simulink model "uav_ue4_depth_imaging"  (R2021b)
settings: Solver=VariableStepAuto  StartTime=0.0  StopTime=10.0  RelTol=1e-3
libraries: visionsinks x3, sim3dcameralib x1, sim3dlib x1, uavsim3dlib x1, simulink x1
settings Model: Creator=The MathWorks, Inc.  LastModifiedBy=The MathWorks, Inc.
settings SolverCC: AlgebraicLoopSolver=TrustRegion
settings DebuggingCC: SFMachineParentedDataDiag=warning

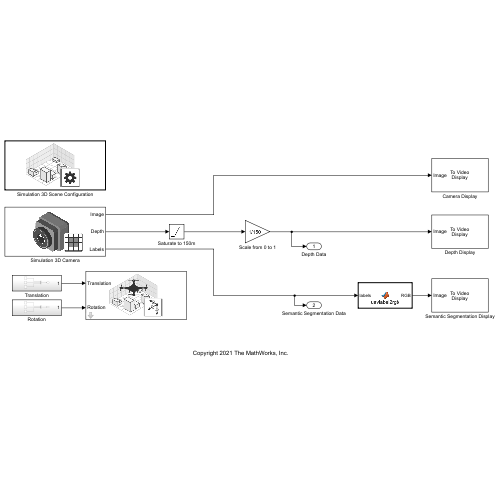
[thumbnail: Simulink's stored preview of the top-level diagram]
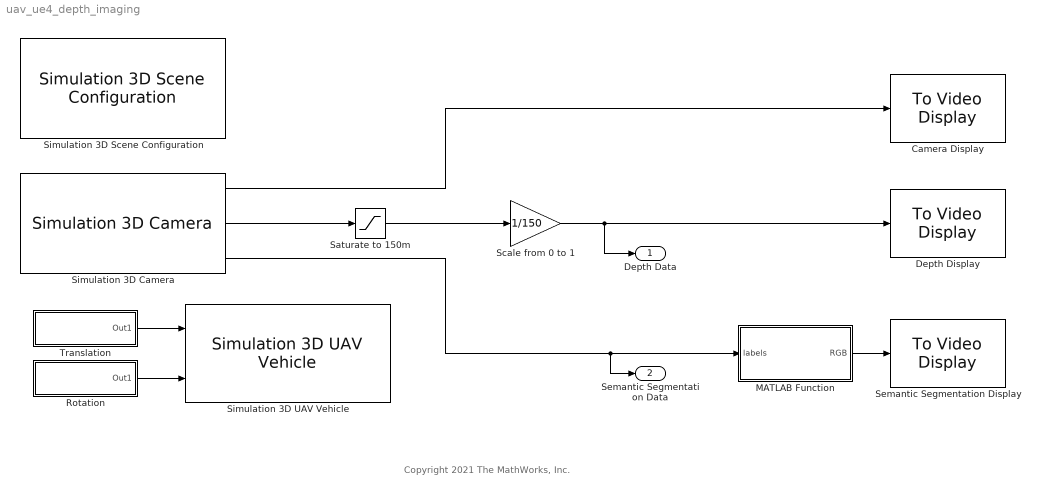
== system uav_ue4_depth_imaging ==
  note: Copyright 2021 The MathWorks, Inc.
  Camera Display : visionsinks/To Video Display  windowSizeMode=Normal  openAtMdlStart=on  fullScreen=off  videoWindowX=3778  videoWindowY=476  saveWindowSize=off  videoWindowWidth=1280  videoWindowHeight=720  inputColorFormat=RGB  inputType=Obsolete  imagePorts=One multidimensional signal  OutputDevice=On-screen video monitor  dataOrg=Column-major  isWindowOpen=off
  Depth Display : visionsinks/To Video Display  windowSizeMode=Normal  openAtMdlStart=on  fullScreen=off  videoWindowX=2800  videoWindowY=206  saveWindowSize=off  videoWindowWidth=1280  videoWindowHeight=720  inputColorFormat=RGB  inputType=Obsolete  imagePorts=One multidimensional signal  OutputDevice=On-screen video monitor  dataOrg=Column-major  isWindowOpen=off
  MATLAB Function : MATLAB Function  TreatAsAtomicUnit=on
  Rotation : Subsystem
  Saturate to 150m : Saturate  UpperLimit=150  LowerLimit=0
  Scale from 0 to 1 : Gain  Gain=1/150
  Semantic Segmentation Display : visionsinks/To Video Display  windowSizeMode=Normal  openAtMdlStart=on  fullScreen=off  videoWindowX=2682  videoWindowY=595  saveWindowSize=off  videoWindowWidth=1280  videoWindowHeight=720  inputColorFormat=RGB  inputType=Obsolete  imagePorts=One multidimensional signal  OutputDevice=On-screen video monitor  dataOrg=Column-major  isWindowOpen=off
  Simulation 3D Camera : sim3dcameralib/Simulation 3D Camera  Priority=1  sensorTag=Sim3dSensor1  sensorId=1  sensorName=Sim3dSensor1  vehTagList={'Scene Origin';'SimulinkVehicle1'}  vehTag=SimulinkVehicle1  mountLoc=Origin  offsetFlag=on  tmountOffset=[0.2, 0, 0]  extTmount=off  rmountOffset=[0, 0, 0]  extRmount=off  FocalLength=[1109, 1109]  OpticalCenter=[640, 360]  ImageSize=[720, 1280]  RadialDistortion=[0, 0]  TangentialDistortion=[0, 0]  SensorSkew=0  DepthOutportEnabled=on  SemanticOutportEnabled=on  TransformOutportEnabled=off  SampleTime=-1  mountPoint=[0.2 0 0]  mountOrientation=[0 0 0]  aMode=4  ID=1
      settings: SourceProductBaseCode=AE,DR,UV,VE
  Simulation 3D Scene Configuration : sim3dlib/Simulation 3D Scene Configuration  Priority=0  ProjectFormat_internal=Default Scenes  ProjectFormat=Default Scenes  SceneDesc=US city block  ProjectName=B:\matlab\toolbox\shared\sim3d_projects\automotive_project\UE4\WindowsNoEditor\VehicleSimulation.exe  ScenePath=/Game/Maps/USCityBlock  vehTagList={'Scene Origin';'SimulinkVehicle1'}  vehTag=Scene Origin  OpVisEn=off  Ts=1/60  EnableWindow=on  EnableWeather=off  SunAltitude=40.0  SunAzimuth=90  clouds=10  wind=1  fog=0  rain=0  sensorTag=MainCamera1  sensorId=1  sensorName=MainCamera1  mountLoc=Origin  offsetFlag=off  tmountOffset=[0, 0, 0]  rmountOffset=[0, 0, 0]  HorizontalResolution=1280  VerticalResolution=720  HorizontalFOV=60  mountPoint=[0 0 0]  mountOrientation=[0 0 0]  aMode=4  ID=1
      settings: SourceProductBaseCode=AE,DR,UV,VE
  Simulation 3D UAV Vehicle : uavsim3dlib/Simulation 3D UAV Vehicle  Priority=-1  Mesh=Quadrotor  MeshPath=/MathWorksUAVContent/UAVs/HexaRotorUAV/HexaRotor.HexaRotor  Color=Black  ActorName=SimulinkVehicle1  InitialTranslation=[0 0 10]  InitialRotation=[0 0 0]  SampleTime=-1  ActorType=SimulinkVehicle  ID=1  aMode=4  ActorTag=SimulinkVehicle1
      settings: SourceProductBaseCode=UV
  Translation : Subsystem
  Depth Data : Outport
  Semantic Segmentation Data : Outport  Port=2
  wires:
  Saturate to 150m/1 -> Scale from 0 to 1/1
  Simulation 3D Camera/2 -> Saturate to 150m/1
  Simulation 3D Camera/3 -> Semantic Segmentation Data/1, MATLAB Function/1(labels)
  Translation/1(Out1) -> Simulation 3D UAV Vehicle/1
  Rotation/1(Out1) -> Simulation 3D UAV Vehicle/2
  MATLAB Function/1(RGB) -> Semantic Segmentation Display/1
  Scale from 0 to 1/1 -> Depth Data/1, Depth Display/1
  Simulation 3D Camera/1 -> Camera Display/1

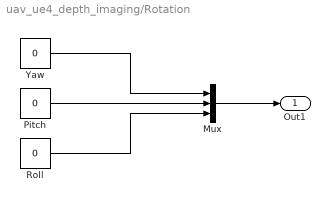
== system uav_ue4_depth_imaging/Rotation ==
  Mux : Mux  Inputs=3
  Pitch : Constant  Value=0
  Roll : Constant  Value=0
  Yaw : Constant  Value=0
  Out1 : Outport
  wires:
  Mux/1 -> Out1/1
  Roll/1 -> Mux/3
  Pitch/1 -> Mux/2
  Yaw/1 -> Mux/1

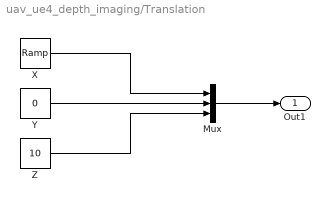
== system uav_ue4_depth_imaging/Translation ==
  Mux : Mux  Inputs=3
  X : simulink/Sources/Ramp  slope=2  start=0  InitialOutput=0
  Y : Constant  Value=0
  Z : Constant  Value=10
  Out1 : Outport
  wires:
  Mux/1 -> Out1/1
  Z/1 -> Mux/3
  Y/1 -> Mux/2
  X/1 -> Mux/1

== matlab function uav_ue4_depth_imaging/MATLAB Function ==
  data: labels input; RGB output
function RGB = uavlabel2rgb(labels)
% Convert semantic segmentation map captured during 3D simulation to RGB
% color image.

% Declare label2rgb function.
coder.extrinsic('label2rgb');

% Preallocate memory for RGB matrix.
RGB = coder.nullcopy(zeros(size(labels,1),size(labels,2),3,class(labels)));

% Define colormap using 3D simulation label IDs.
cmap = sim3dColormap;

% Convert labels to RGB color image.
RGB = label2rgb(labels, cmap);
